simulink model "mainCameraLiDAR"  (R2024b)
settings: Solver=FixedStepDiscrete  StartTime=0  StopTime=70  FixedStep=0.025  RelTol=1e-3
libraries: VDriveToolbox x18
settings Model: Creator=tatsu  LastModifiedBy=INOUE MASATO
settings SolverCC: AlgebraicLoopSolver=TrustRegion
settings DebuggingCC: UnconnectedInputMsg=warning  UnconnectedOutputMsg=warning  UnconnectedLineMsg=warning
settings ModelReferenceCC: EnableRefExpFcnMdlSchedulingChecks=on
settings RTWCC: GPUComputeCapability=3.5

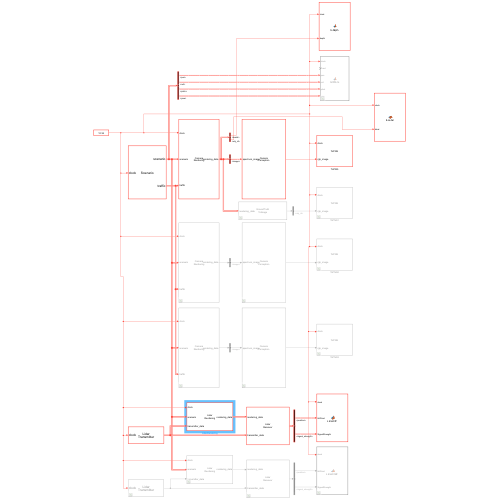
[thumbnail: Simulink's stored preview of the top-level diagram]
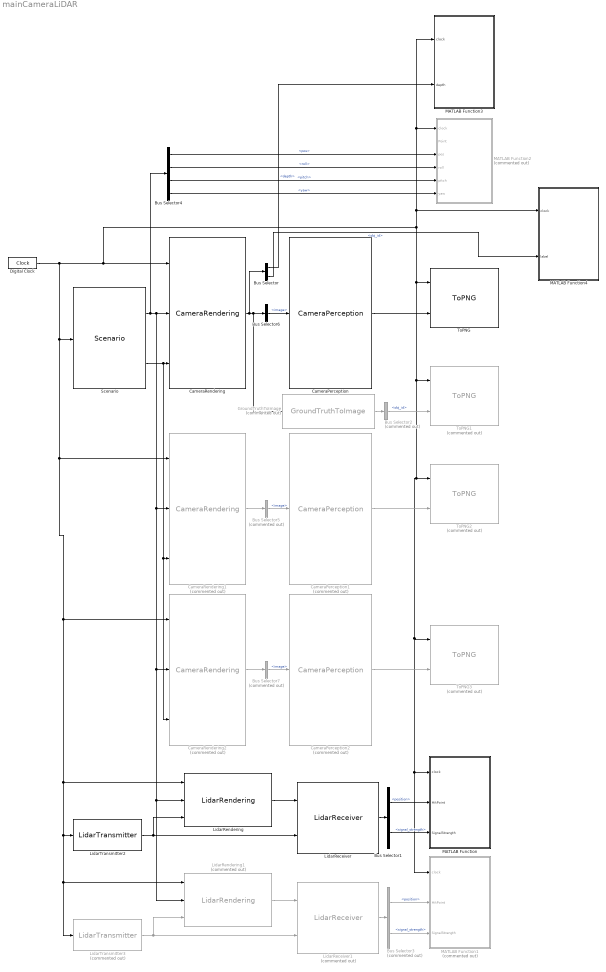
== system mainCameraLiDAR ==
  Bus Selector : BusSelector  OutputSignals=depth,obj_id
  Bus Selector1 : BusSelector  OutputSignals=position,signal_strength
  Bus Selector2 : BusSelector  Commented=on  OutputSignals=obj_id
  Bus Selector3 : BusSelector  Commented=on  OutputSignals=position,signal_strength
  Bus Selector4 : BusSelector  OutputSignals=pos,roll,pitch,yaw
  Bus Selector5 : BusSelector  Commented=on  OutputSignals=image
  Bus Selector6 : BusSelector  OutputSignals=image
  Bus Selector7 : BusSelector  Commented=on  OutputSignals=image
  CameraPerception : VDriveToolbox/Cameras/CameraPerception  PerEControl=Auto  PerUBound=10.0  PerLBound=0.0  PerIsGamma="\"on\""
      settings: SourceProductName=V-Drive Toolbox
  CameraPerception1 : VDriveToolbox/Cameras/CameraPerception  Commented=on  PerEControl=Auto  PerUBound=10.0  PerLBound=0.0  PerIsGamma="\"on\""
      settings: SourceProductName=V-Drive Toolbox
  CameraPerception2 : VDriveToolbox/Cameras/CameraPerception  Commented=on  PerEControl=Auto  PerUBound=10.0  PerLBound=0.0  PerIsGamma="\"on\""
      settings: SourceProductName=V-Drive Toolbox
  CameraRendering : VDriveToolbox/Cameras/CameraRendering  SubConfigFile="\"myconfig/camera_rendering_sample2.json\""  SubScenarioXML="\"scenario/dataset_3/dataset_making3_csv.xml\""  SubScenarioID="\"scenario_1\""  SubSensorID="\"camera_5\""  SubSampleTime=-1
      settings: SourceProductName=V-Drive Toolbox
  CameraRendering1 : VDriveToolbox/Cameras/CameraRendering  Commented=on  SubConfigFile="\"myconfig/camera_rendering_sample2.json\""  SubScenarioXML="\"scenario/manhole/man-hole_csv.xml\""  SubScenarioID="\"scenario_1\""  SubSensorID="\"camera_right\""  SubSampleTime=-1
      settings: SourceProductName=V-Drive Toolbox
  CameraRendering2 : VDriveToolbox/Cameras/CameraRendering  Commented=on  SubConfigFile="\"myconfig/camera_rendering_sample2.json\""  SubScenarioXML="\"scenario/manhole/man-hole_csv.xml\""  SubScenarioID="\"scenario_1\""  SubSensorID="\"camera_left\""  SubSampleTime=-1
      settings: SourceProductName=V-Drive Toolbox
  Digital Clock : DigitalClock  SampleTime=0.025
  GroundTruthToImage : VDriveToolbox/Cameras/GroundTruthToImage  Commented=on
      settings: SourceProductName=V-Drive Toolbox
  LidarReceiver : VDriveToolbox/Lidars/LidarReceiver  SubsignalRange=[-100 -19]  SubsampleTime=-1
      settings: SourceProductName=V-Drive Toolbox
  LidarReceiver1 : VDriveToolbox/Lidars/LidarReceiver  Commented=on  SubsignalRange=[-100 -19]  SubsampleTime=-1
      settings: SourceProductName=V-Drive Toolbox
  LidarRendering : VDriveToolbox/Lidars/LidarRendering  SubConfigFile="\"myconfig/os-1-64_rendering.json\""  SubScenarioXML="\"scenario/dataset_3/dataset_making3_csv.xml\""  SubScenarioID="\"scenario_1\""  SubSensorID="\"lidar_3\""  SubSampleTime=-1
      settings: SourceProductName=V-Drive Toolbox
  LidarRendering1 : VDriveToolbox/Lidars/LidarRendering  Commented=on  SubConfigFile="\"myconfig/os-1-128_rendering.json\""  SubScenarioXML="\"scenario/dataset_1/sample_loop_output.xml\""  SubScenarioID="\"scenario_1\""  SubSensorID="\"lidar_2\""  SubSampleTime=-1
      settings: SourceProductName=V-Drive Toolbox
  LidarTransmitter2 : VDriveToolbox/Lidars/LidarTransmitter  SuboperationFreq=40  SubazimuthAngle=[-pi pi 0.006135923151543]  SubzenithAngle=[1.178097245 1.963495408 0.01227185]  SubmaxRayNum=66500  SubsampleTime=-1
      settings: SourceProductName=V-Drive Toolbox
  LidarTransmitter3 : VDriveToolbox/Lidars/LidarTransmitter  Commented=on  SuboperationFreq=20  SubazimuthAngle=[-pi pi 0.006135923]  SubzenithAngle=[1.178097245 1.963495408 0.00613592315]  SubmaxRayNum=133000  SubsampleTime=-1
      settings: SourceProductName=V-Drive Toolbox
  MATLAB Function : MATLAB Function  TreatAsAtomicUnit=on
  MATLAB Function1 : MATLAB Function  Commented=on  TreatAsAtomicUnit=on
  MATLAB Function2 : MATLAB Function  Commented=on  TreatAsAtomicUnit=on
  MATLAB Function3 : MATLAB Function  TreatAsAtomicUnit=on
  MATLAB Function4 : MATLAB Function  TreatAsAtomicUnit=on
  Scenario : VDriveToolbox/Scenarios/Scenario  SubScenarioXML="\"scenario/dataset_3/dataset_making3_csv.xml\""  SubScenarioID="\"scenario_1\""
      settings: SourceProductName=V-Drive Toolbox
  ToPNG : VDriveToolbox/Cameras/ToPNG   file_name="\"image\""  dir="\"image_front\""
      settings: SourceProductName=V-Drive Toolbox
  ToPNG1 : VDriveToolbox/Cameras/ToPNG   Commented=on  file_name="\"label\""  dir="\"gt_label\""
      settings: SourceProductName=V-Drive Toolbox
  ToPNG2 : VDriveToolbox/Cameras/ToPNG   Commented=on  file_name="\"image\""  dir="\"image_right\""
      settings: SourceProductName=V-Drive Toolbox
  ToPNG3 : VDriveToolbox/Cameras/ToPNG   Commented=on  file_name="\"image\""  dir="\"image_left\""
      settings: SourceProductName=V-Drive Toolbox
  wires:
  Scenario/1 -> Bus Selector4/1, CameraRendering/2, CameraRendering1/2, CameraRendering2/2, LidarRendering/2, LidarRendering1/2
  Scenario/2 -> CameraRendering2/3, CameraRendering1/3, CameraRendering/3
  CameraPerception/1 -> ToPNG/2
  CameraRendering/1 -> Bus Selector/1, Bus Selector6/1, GroundTruthToImage/1
  Digital Clock/1 -> MATLAB Function4/1(clock), MATLAB Function3/1(clock), MATLAB Function2/1(clock), ToPNG/1, ToPNG3/1, MATLAB Function/1(clock), MATLAB Function1/1(clock), ToPNG2/1, ToPNG1/1, CameraRendering/1, CameraRendering1/1, CameraRendering2/1, LidarTransmitter2/1, LidarTransmitter3/1, LidarRendering1/1, LidarRendering/1, Scenario/1
  LidarRendering/1 -> LidarReceiver/1
  LidarReceiver/1 -> Bus Selector1/1
  Bus Selector1/2 -> MATLAB Function/3(SignalStrength)  "<signal_strength>"
  Bus Selector1/1 -> MATLAB Function/2(HitPoint)  "<position>"
  LidarTransmitter2/1 -> LidarRendering/3, LidarReceiver/2
  GroundTruthToImage/1 -> Bus Selector2/1
  Bus Selector2/1 -> ToPNG1/2  "<obj_id>"
  Bus Selector3/2 -> MATLAB Function1/3(SignalStrength)  "<signal_strength>"
  LidarTransmitter3/1 -> LidarRendering1/3, LidarReceiver1/2
  LidarReceiver1/1 -> Bus Selector3/1
  Bus Selector3/1 -> MATLAB Function1/2(HitPoint)  "<position>"
  LidarRendering1/1 -> LidarReceiver1/1
  Bus Selector/1 -> MATLAB Function3/2(depth)  "<depth>"
  Bus Selector4/1 -> MATLAB Function2/3(pos)  "<pos>"
  Bus Selector4/2 -> MATLAB Function2/4(roll)  "<roll>"
  Bus Selector4/3 -> MATLAB Function2/5(pitch)  "<pitch>"
  Bus Selector4/4 -> MATLAB Function2/6(yaw)  "<yaw>"
  CameraRendering1/1 -> Bus Selector5/1
  Bus Selector6/1 -> CameraPerception/1  "<image>"
  Bus Selector5/1 -> CameraPerception1/1  "<image>"
  CameraPerception1/1 -> ToPNG2/2
  Bus Selector7/1 -> CameraPerception2/1  "<image>"
  CameraRendering2/1 -> Bus Selector7/1
  CameraPerception2/1 -> ToPNG3/2
  Bus Selector/2 -> MATLAB Function4/2(label)  "<obj_id>"

== matlab function mainCameraLiDAR/MATLAB Function1 ==
  data: clock input; HitPoint input; SignalStrength input
function LidarXYZ2(clock,HitPoint,SignalStrength)
    lidar_name = 'front-lidar';
    save_dir = "pcd_"+lidar_name;

    coder.extrinsic('func_LidarXYZMap_front');
    func_LidarXYZMap_front(lidar_name,clock,HitPoint,SignalStrength,save_dir);
    
end

== matlab function mainCameraLiDAR/MATLAB Function2 ==
  data: clock input; Point input; pos input; roll input; pitch input; yaw input
function GtPoints(clock,Point,pos,roll,pitch,yaw)
    points_name = 'gtpoints';

    coder.extrinsic('func_getGtPoints');
    func_getGtPoints(points_name,clock,Point,pos,roll,pitch,yaw);
    
end

== matlab function mainCameraLiDAR/MATLAB Function3 ==
  data: clock input; depth input
function toDepth(clock,depth)
    scale_factor = 20;
    save_dir = 'gt_depth';

    coder.extrinsic('func_getGtDepth');
    func_getGtDepth(clock,depth,scale_factor,save_dir);
    
end

== matlab function mainCameraLiDAR/MATLAB Function4 ==
  data: clock input; label input
function toLabel(clock,label)
    save_dir = 'gt_label';

    coder.extrinsic('func_getGtLabel');
    func_getGtLabel(clock,label,save_dir);
    
end

== matlab function mainCameraLiDAR/MATLAB Function ==
  data: clock input; HitPoint input; SignalStrength input
function LidarXYZ(clock,HitPoint,SignalStrength)
    lidar_name = 'roof-lidar';
    save_dir = "pcd_"+lidar_name;

    coder.extrinsic('func_LidarXYZMap_roof');
    func_LidarXYZMap_roof(lidar_name,clock,HitPoint,SignalStrength,save_dir);
    
end
